simulink model "Lane Following and Object detection Simulink Model"  (R2024b)
settings: Solver=FixedStepDiscrete  StartTime=0.0  StopTime=10.0  RelTol=1e-3
undefined symbols (not defined in the file or in its folder): driving
libraries: drivingscenarioandsensors x6
(part 1 of 2)
settings Model: Creator=Sohan  LastModifiedBy=Sohan

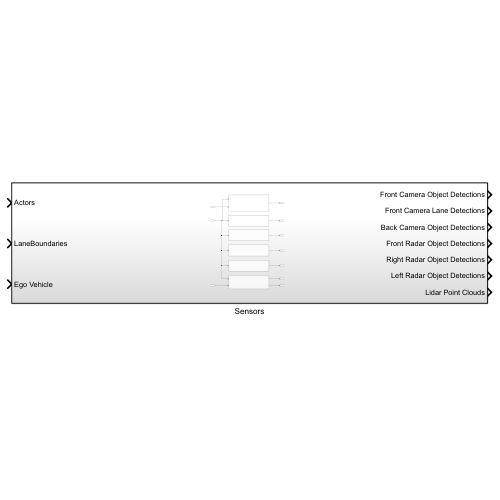
[thumbnail: Simulink's stored preview of the top-level diagram]
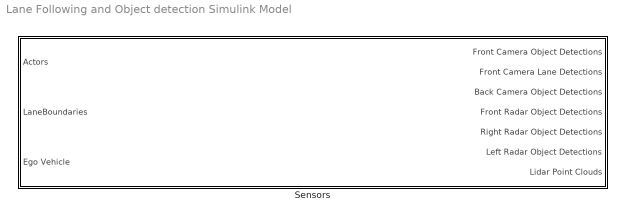
== system Lane Following and Object detection Simulink Model ==
  Sensors : Subsystem
